simulink model "PVESsystem"  (R2024a)
settings: Solver=FixedStepDiscrete  StartTime=0.0  StopTime=4  FixedStep=1e-7  MaxStep=1e-6  RelTol=1e-3
libraries: spsSeriesRLCBranchLib x11, spsMultimeterLib x4, spsDiodeLib x2, spsMosfetLib x2, slpidlib x2, eePwmGenerator x2, spsVoltageMeasurementLib x2, spsCurrentMeasurementLib x1, spsDCVoltageSourceLib x1, spsPVArrayLib x1, sps_lib x1
settings Model: Creator=admin  LastModifiedBy=ZE
settings SolverCC: AllowMultiTaskInputOutput=on
settings ModelReferenceCC: EnableParallelModelReferenceBuilds=on
settings SFSimCC: SimTargetLang=C++  GPUAcceleration=on  SimDLTargetLibrary=cudnn

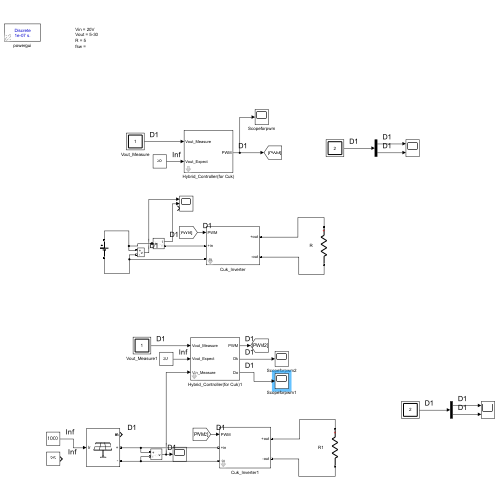
[thumbnail: Simulink's stored preview of the top-level diagram]
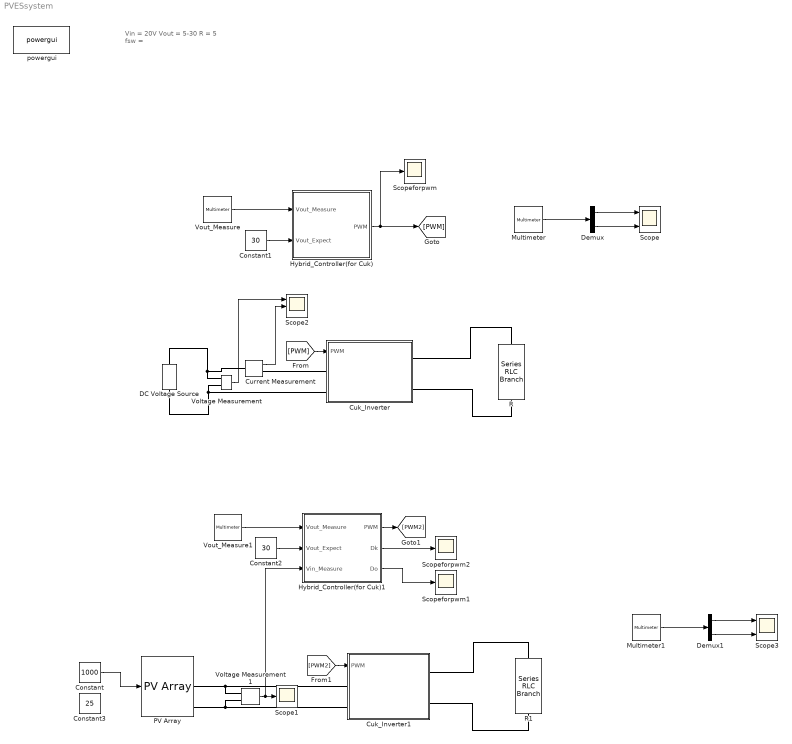
== system PVESsystem ==
  note: Vin = 20V
      | Vout = 5-30
      | R = 5
      | fsw =
  Constant : Constant  Value=1000
  Constant1 : Constant  Value=30
  Constant2 : Constant  Value=30
  Constant3 : Constant  Value=25
  Cuk_Inverter : Subsystem  mask{Vin=30, Vout_Expect=40, Fsw=100e3, detaIL1=0.1, detaIL2=0.1, detaUC1=0.1, detaUC2=0.1}
      mask prompts: Fsw "Switch Frequency"; detaIL1 "电感纹波"; detaIL2 "电感纹波"; detaUC1 "电压纹波"; detaUC2 "电压纹波"
      mask DialogControl ParameterGroupVar Prompt: 参数
  Cuk_Inverter1 : Subsystem  mask{Vin=30, Vout_Expect=40, Fsw=100e3, detaIL1=0.1, detaIL2=0.1, detaUC1=0.1, detaUC2=0.1}
      mask prompts: Fsw "Switch Frequency"; detaIL1 "电感纹波"; detaIL2 "电感纹波"; detaUC1 "电压纹波"; detaUC2 "电压纹波"
      mask DialogControl ParameterGroupVar Prompt: 参数
  Current Measurement : spsCurrentMeasurementLib/Current Measurement  PhasorSimulation=off  OutputType=Complex  PSBequivalent=0
  DC Voltage Source : spsDCVoltageSourceLib/DC Voltage Source  Amplitude=30  Measurements=None
  Demux : Demux  Outputs=2
  Demux1 : Demux  Outputs=2
  Hybrid_Controller(for Cuk) : Subsystem  mask{Vout_Expect=20, Vin=30, Fsw=100e3}
      mask prompts: Fsw "switch frequency"
      mask DialogControl ParameterGroupVar Prompt: 参数
  Hybrid_Controller(for Cuk)1 : Subsystem  mask{Vout_Expect=20, Vin=30, Fsw=100e3}
      mask prompts: Fsw "switch frequency"
      mask DialogControl ParameterGroupVar Prompt: 参数
  Multimeter : spsMultimeterLib/Multimeter  L=4  sel=[1 3]  yselected={}  Gain=[1 1]  OutputType=Complex  PlotAtSimulationStop=off  PhasorSimulation=off
  Multimeter1 : spsMultimeterLib/Multimeter  L=4  sel=[2 4]  yselected={}  Gain=[1 1]  OutputType=Complex  PlotAtSimulationStop=off  PhasorSimulation=off
  PV Array : spsPVArrayLib/PV Array  Npar=20  Nser=1  PlotType=array @ 1000 W/m2 & specified temperatures  S_vec="[ 1000  500  100 ]"  Temp_C_vec="[ 45 25  ]"  ModuleName=User-defined  PlotWhenSelected=off  Pm=213.15  Ncell=60  Voc=36.3  Isc=7.84  Vm=29  Im=7.35  beta_Voc_pc=-0.36099  alpha_Isc_pc=0.102  beta_Voc=-0.13104  alpha_Isc=0.0079968  IL=7.8654  I0=2.9273e-10  nI=0.98119  Rsh=313.0553  Rs=0.39381  RobustModel=on  RobustCellTemperature=25  BAL=on  Tc=1e-6  Tfilter=5e-5
  R : spsSeriesRLCBranchLib/Series RLC Branch  LConnTagsString=__new0  RConnTagsString=__new0  BranchType=R  Resistance=5  Inductance=1e-3  SetiL0=off  InitialCurrent=0  Capacitance=1e-6  Setx0=off  InitialVoltage=0  Measurements=Branch voltage and current
  R1 : spsSeriesRLCBranchLib/Series RLC Branch  LConnTagsString=__new0  RConnTagsString=__new0  BranchType=R  Resistance=5  Inductance=1e-3  SetiL0=off  InitialCurrent=0  Capacitance=1e-6  Setx0=off  InitialVoltage=0  Measurements=Branch voltage and current
  Scope : Scope  NumInputPorts=2
  Scope1 : Scope
  Scope2 : Scope  NumInputPorts=3
  Scope3 : Scope  NumInputPorts=2
  Scopeforpwm : Scope
  Scopeforpwm1 : Scope
  Scopeforpwm2 : Scope
  Voltage Measurement : spsVoltageMeasurementLib/Voltage Measurement  PhasorSimulation=off  OutputType=Complex  PSBequivalent=0
  Voltage Measurement1 : spsVoltageMeasurementLib/Voltage Measurement  PhasorSimulation=off  OutputType=Complex  PSBequivalent=0
  Vout_Measure : spsMultimeterLib/Multimeter  L=4  sel=1  yselected={}  Gain=1  OutputType=Complex  PlotAtSimulationStop=off  PhasorSimulation=off
  Vout_Measure1 : spsMultimeterLib/Multimeter  L=4  sel=2  yselected={}  Gain=1  OutputType=Complex  PlotAtSimulationStop=off  PhasorSimulation=off
  powergui : sps_lib/powergui  Priority=1  SimulationMode=Discrete  SampleTime=1e-7  frequency=60  Iterations=50  frequencyindice=0  Pbase=100e6  ErrMax=1e-4  UnitsV=kV  UnitsW=MW  buscounter=0  FunctionMessages=off  echomessages=off  EnableUseOfTLC=off  CurrentSourceSwitches=off  DisableSnubberDevices=off  DisableRonSwitches=off  DisableVfSwitches=off  DisplayEquations=off  AutomaticDiscreteSolvers=off  SolverType=Tustin/Backward Euler (TBE)  Interpol=off  ExternalGateDelay=off  methode=off  Ts=100  x0status=blocks  SPID=on  SwTol=0  HookPort=off  NonlinearTolerance=1e-4  nMaxIteration=100  ContinueOnMaxIteration=off  RestoreLinks=warning  ResistiveCurrentMeasurement=off  Frange=[0:2:500]  Ylog=off  Xlog=on  ShowGrid=off  save=off  variable=ZData  structure=0  ZoomFFT=off  StartTime=0.0  cycles=1  DisplayStyle=1  fundamental=60  FreqAxis=off  MaxFrequency=1000  frequencyindicesteady=1  RmsSteady=1  display=off
  wires:
  Vout_Measure/1 -> Hybrid_Controller(for Cuk)/1(Vout_Measure)
  Hybrid_Controller(for Cuk)/1(PWM) -> Scopeforpwm/1, [PWM]
  [PWM] -> Cuk_Inverter/1(PWM)
  Voltage Measurement/1 -> Scope2/1
  Current Measurement/1 -> Scope2/2
  Constant1/1 -> Hybrid_Controller(for Cuk)/2(Vout_Expect)
  Multimeter/1 -> Demux/1
  Demux/1 -> Scope/1
  Demux/2 -> Scope/2
  [PWM2] -> Cuk_Inverter1/1(PWM)
  Constant2/1 -> Hybrid_Controller(for Cuk)1/2(Vout_Expect)
  Vout_Measure1/1 -> Hybrid_Controller(for Cuk)1/1(Vout_Measure)
  Hybrid_Controller(for Cuk)1/1(PWM) -> [PWM2]
  Demux1/2 -> Scope3/2
  Demux1/1 -> Scope3/1
  Multimeter1/1 -> Demux1/1
  Constant/1 -> PV Array/1
  Voltage Measurement1/1 -> Hybrid_Controller(for Cuk)1/3(Vin_Measure), Scope1/1
  Hybrid_Controller(for Cuk)1/2(Dk) -> Scopeforpwm2/1
  Hybrid_Controller(for Cuk)1/3(Do) -> Scopeforpwm1/1
  connections:
  R/LConn1 -- Cuk_Inverter/RConn1
  R/RConn1 -- Cuk_Inverter/RConn2
  Current Measurement/LConn1 -- DC Voltage Source/RConn1 -- Voltage Measurement/LConn1
  Voltage Measurement/LConn2 -- DC Voltage Source/LConn1 -- Cuk_Inverter/LConn2
  Current Measurement/RConn1 -- Cuk_Inverter/LConn1
  Cuk_Inverter1/LConn1 -- Voltage Measurement1/LConn1 -- PV Array/RConn1
  PV Array/RConn2 -- Voltage Measurement1/LConn2 -- Cuk_Inverter1/LConn2
  R1/RConn1 -- Cuk_Inverter1/RConn2
  R1/LConn1 -- Cuk_Inverter1/RConn1

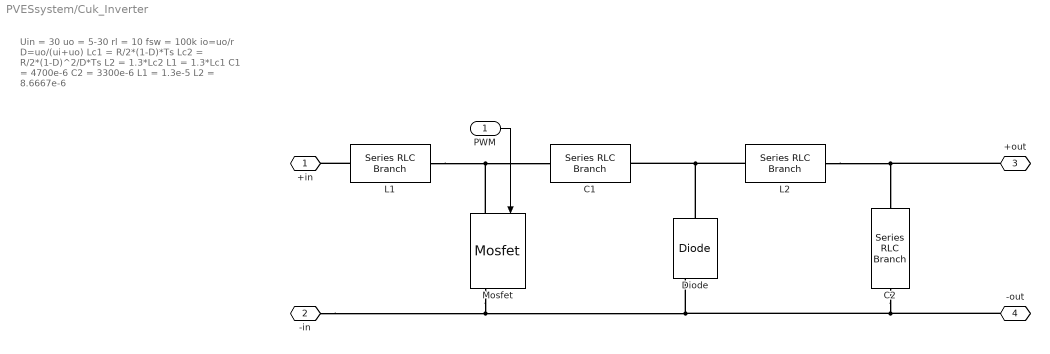
== system PVESsystem/Cuk_Inverter ==
  note: Uin = 30
      | uo = 5-30
      | rl = 10
      | fsw = 100k
      | io=uo/r
      |
      | D=uo/(ui+uo)
      | Lc1 = R/2*(1-D)*Ts
      | Lc2 = R/2*(1-D)^2/D*Ts
      | L2 = 1.3*Lc2
      | L1 = 1.3*Lc1
      | C1 = 4700e-6
      | C2 = 3300e-6
      |
      | L1 = 1.3e-5
      | L2 = 8.6667e-6
  PWM : Inport
  C1 : spsSeriesRLCBranchLib/Series RLC Branch  LConnTagsString=__new0  RConnTagsString=__new0  BranchType=C  Resistance=1  Inductance=1e-3  SetiL0=off  InitialCurrent=0  Capacitance=0.0047  Setx0=off  InitialVoltage=0  Measurements=None
  C2 : spsSeriesRLCBranchLib/Series RLC Branch  LConnTagsString=__new0  RConnTagsString=__new0  BranchType=C  Resistance=1  Inductance=1e-3  SetiL0=off  InitialCurrent=0  Capacitance=0.0033  Setx0=off  InitialVoltage=0  Measurements=None
  Diode : spsDiodeLib/Diode  Ron=0.001  Lon=0  Vf=0.8  IC=0  UseSnubber=0  Rs=500  Cs=250e-9  Measurements=on
  L1 : spsSeriesRLCBranchLib/Series RLC Branch  LConnTagsString=__new0  RConnTagsString=__new0  BranchType=L  Resistance=1  Inductance=1.3e-5  SetiL0=off  InitialCurrent=0  Capacitance=1e-6  Setx0=off  InitialVoltage=0  Measurements=None
  L2 : spsSeriesRLCBranchLib/Series RLC Branch  LConnTagsString=__new0  RConnTagsString=__new0  BranchType=L  Resistance=1  Inductance=8.6667e-6  SetiL0=off  InitialCurrent=0  Capacitance=1e-6  Setx0=off  InitialVoltage=0  Measurements=None
  Mosfet : spsMosfetLib/Mosfet  Ron=0.1  Lon=0  Rd=0.01  Vfd=0  IC=0  Rs=1e5  Cs=inf  Measurements=on
  +in : PMIOPort  Side=Left
  -in : PMIOPort  Port=2  Side=Left
  +out : PMIOPort  Port=3  Side=Right
  -out : PMIOPort  Port=4  Side=Right
  wires:
  PWM/1 -> Mosfet/1
  connections:
  L2/RConn1 -- +out/RConn1 -- C2/LConn1
  L2/LConn1 -- Diode/LConn1 -- C1/RConn1
  L1/LConn1 -- +in/RConn1
  L1/RConn1 -- Mosfet/LConn1 -- C1/LConn1
  Mosfet/RConn1 -- -in/RConn1 -- -out/RConn1 -- C2/RConn1 -- Diode/RConn1

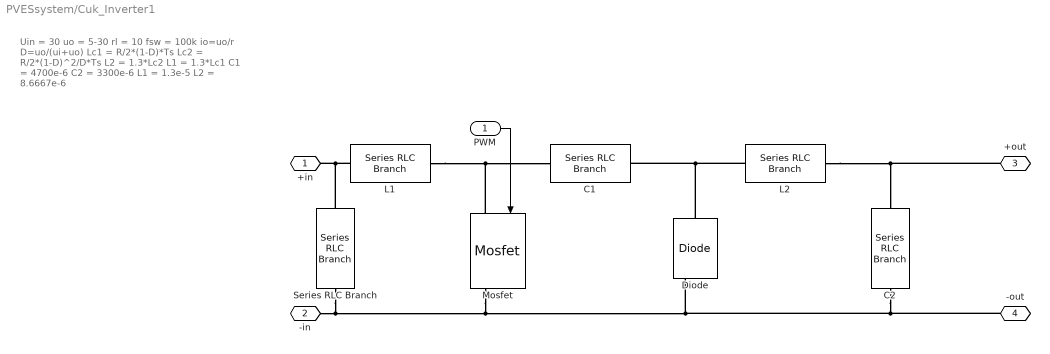
== system PVESsystem/Cuk_Inverter1 ==
  note: Uin = 30
      | uo = 5-30
      | rl = 10
      | fsw = 100k
      | io=uo/r
      |
      | D=uo/(ui+uo)
      | Lc1 = R/2*(1-D)*Ts
      | Lc2 = R/2*(1-D)^2/D*Ts
      | L2 = 1.3*Lc2
      | L1 = 1.3*Lc1
      | C1 = 4700e-6
      | C2 = 3300e-6
      |
      | L1 = 1.3e-5
      | L2 = 8.6667e-6
  PWM : Inport
  C1 : spsSeriesRLCBranchLib/Series RLC Branch  LConnTagsString=__new0  RConnTagsString=__new0  BranchType=C  Resistance=1  Inductance=1e-3  SetiL0=off  InitialCurrent=0  Capacitance=0.0047  Setx0=off  InitialVoltage=0  Measurements=None
  C2 : spsSeriesRLCBranchLib/Series RLC Branch  LConnTagsString=__new0  RConnTagsString=__new0  BranchType=C  Resistance=1  Inductance=1e-3  SetiL0=off  InitialCurrent=0  Capacitance=0.0033  Setx0=off  InitialVoltage=0  Measurements=None
  Diode : spsDiodeLib/Diode  Ron=0.001  Lon=0  Vf=0.8  IC=0  UseSnubber=0  Rs=500  Cs=250e-9  Measurements=on
  L1 : spsSeriesRLCBranchLib/Series RLC Branch  LConnTagsString=__new0  RConnTagsString=__new0  BranchType=L  Resistance=1  Inductance=1.3e-5  SetiL0=off  InitialCurrent=0  Capacitance=1e-6  Setx0=off  InitialVoltage=0  Measurements=None
  L2 : spsSeriesRLCBranchLib/Series RLC Branch  LConnTagsString=__new0  RConnTagsString=__new0  BranchType=L  Resistance=1  Inductance=8.6667e-6  SetiL0=off  InitialCurrent=0  Capacitance=1e-6  Setx0=off  InitialVoltage=0  Measurements=None
  Mosfet : spsMosfetLib/Mosfet  Ron=0.1  Lon=0  Rd=0.01  Vfd=0  IC=0  Rs=1e5  Cs=inf  Measurements=on
  Series RLC Branch : spsSeriesRLCBranchLib/Series RLC Branch  LConnTagsString=__new0  RConnTagsString=__new0  BranchType=C  Resistance=1  Inductance=1e-3  SetiL0=off  InitialCurrent=0  Capacitance=1e-6  Setx0=off  InitialVoltage=0  Measurements=None
  +in : PMIOPort  Side=Left
  -in : PMIOPort  Port=2  Side=Left
  +out : PMIOPort  Port=3  Side=Right
  -out : PMIOPort  Port=4  Side=Right
  wires:
  PWM/1 -> Mosfet/1
  connections:
  L2/RConn1 -- +out/RConn1 -- C2/LConn1
  L2/LConn1 -- Diode/LConn1 -- C1/RConn1
  L1/LConn1 -- Series RLC Branch/LConn1 -- +in/RConn1
  L1/RConn1 -- Mosfet/LConn1 -- C1/LConn1
  Mosfet/RConn1 -- -in/RConn1 -- Series RLC Branch/RConn1 -- -out/RConn1 -- C2/RConn1 -- Diode/RConn1

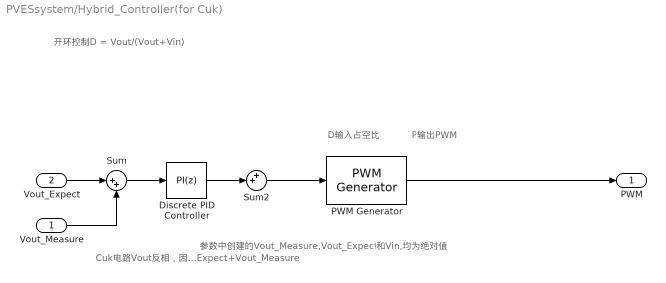
== system PVESsystem/Hybrid_Controller(for Cuk) ==
  note: 开环控制D = Vout/(Vout+Vin)
  note: 参数中创建的Vout_Measure,Vout_Expect和Vin,均为绝对值
  note: Cuk电路Vout反相，因此这里设置为Vout_Expect+Vout_Measure
  note: P输出PWM
  note: D输入占空比
  Vout_Measure : Inport
  Vout_Expect : Inport  Port=2
  Discrete PID Controller : slpidlib/PID Controller  Controller=PI  Form=Parallel  TimeDomain=Discrete-time  UseExternalTs=off  SampleTime=-1  IntegratorMethod=Forward Euler  FilterMethod=Forward Euler  ControllerParametersSource=internal  P=(1/(Vin+1))*10  I=(1/(Vin+1))*5*20  UseKiTs=off  D=0  UseExternalDerivativeSource=off  N=100  UseFilter=on  TunerSelectOption=Transfer Function Based (PID Tuner App)  InitialConditionSource=internal  InitialConditionForIntegrator=0  InitialConditionForFilter=0  DifferentiatorICPrevScaledInput=0  ExternalReset=none  TrackingMode=off  Kt=1  LimitOutput=on  SatLimitsSource=internal  UpperSaturationLimit=0.98  LowerSaturationLimit=0  LinearizeAsGain=off  AntiWindupMode=none  Kb=1  LimitIntegrator=off  UpperIntegratorSaturationLimit=inf  LowerIntegratorSaturationLimit=-inf  POutMin=[]  POutMax=[]  IOutMin=[]  IOutMax=[]  DOutMin=[]  DOutMax=[]  NOutMin=[]  NOutMax=[]  SumOutMin=[]  SumOutMax=[]  SaturationOutMin=[]  SaturationOutMax=[]  PParamMin=[]  PParamMax=[]  IParamMin=[]  IParamMax=[]  DParamMin=[]  DParamMax=[]  NParamMin=[]  NParamMax=[]  KbParamMin=[]  KbParamMax=[]  KtParamMin=[]  KtParamMax=[]  KbOutMin=[]  KbOutMax=[]  KtOutMin=[]  KtOutMax=[]  IntegratorOutMin=[]  IntegratorOutMax=[]  FilterOutMin=[]  FilterOutMax=[]  SumI1OutMin=[]  SumI1OutMax=[]  SumI2OutMin=[]  SumI2OutMax=[]  SumI3OutMin=[]  SumI3OutMax=[]  SumI4OutMin=[]  SumI4OutMax=[]  SumDOutMin=[]  SumDOutMax=[]  DifferentiatorOutMin=[]  DifferentiatorOutMax=[]  FilterDiffOutCoefMin=[]  FilterDiffOutCoefMax=[]  ReciprocalOutMin=[]  ReciprocalOutMax=[]  SumDenOutMin=[]  SumDenOutMax=[]  SumNumOutMin=[]  SumNumOutMax=[]  DivideOutMin=[]  DivideOutMax=[]  UdiffTsProdOutMin=[]  UdiffTsProdOutMax=[]  NTsProdOutMin=[]  NTsProdOutMax=[]  UintegralTsProdOutMin=[]  UintegralTsProdOutMax=[]  UngainTsProdOutMin=[]  UngainTsProdOutMax=[]  ClampingZeroOutDataTypeStr=Inherit: Inherit via back propagation  ClampingZeroOutMin=[]  ClampingZeroOutMax=[]  FilterDenConstantOutDataTypeStr=Inherit: Inherit via back propagation  FilterDenConstantOutMin=[]  FilterDenConstantOutMax=[]  PCopyOutDataTypeStr=Inherit: Inherit via back propagation  PCopyOutMin=[]  PCopyOutMax=[]  NCopyOutDataTypeStr=Inherit: Inherit via back propagation  NCopyOutMin=[]  NCopyOutMax=[]  IntegratorContinuousStateAttributes=''  IntegratorStateMustResolveToSignalObject=off  IntegratorRTWStateStorageClass=Auto  FilterContinuousStateAttributes=''  FilterStateMustResolveToSignalObject=off  FilterRTWStateStorageClass=Auto  ParallelPVariant=InternalParameters  IdealPVariant=Disabled  IVariant=InternalParameters  DVariant=Disabled  IntegratorVariant=Discrete  SatVariant=Enabled  AWVariant=Passthrough  PCopyVariant=Disabled  TRVariant=Disabled  FdbkBlocksVariant=Forward  IdealPFdbkVariant=Disabled  SatFdbkVariant=Disabled  DerivativeFilterVariant=Disabled  NVariant=Disabled  NCopyVariant=Disabled_SignalSpec  FilterICVariant=Disabled  IntegratorICVariant=InternalICs  ExternalResetVariant=Disabled  TRSumVariant=Passthrough  SumFdbkVariant=Disabled  SumVariant=Sum_PI  TsampFilterVariant=InternalTs  TsampNgainVariant=Passthrough  TsampIntegralVariant=Disabled_SignalSpec  ExternalSaturationOutDataTypeStr=Inherit: Same as second input  DerivativeSourceVariant=Disabled
      settings: LibrarySourceBlock=simulink/Discrete/Discrete PID Controller
  PWM Generator : eePwmGenerator/PWM Generator  CarrCount=Up  Tper=1e-5  Tdelay=0  Ts=1e-7
  Sum : Sum  Inputs=|++
  Sum2 : Sum  Inputs=++|
  PWM : Outport
  wires:
  Sum/1 -> Discrete PID Controller/1
  PWM Generator/1 -> PWM/1
  Vout_Expect/1 -> Sum/1
  Vout_Measure/1 -> Sum/2
  Discrete PID Controller/1 -> Sum2/2
  Sum2/1 -> PWM Generator/1

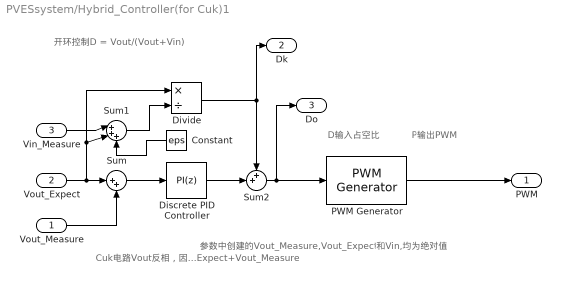
== system PVESsystem/Hybrid_Controller(for Cuk)1 ==
  note: 开环控制D = Vout/(Vout+Vin)
  note: 参数中创建的Vout_Measure,Vout_Expect和Vin,均为绝对值
  note: Cuk电路Vout反相，因此这里设置为Vout_Expect+Vout_Measure
  note: P输出PWM
  note: D输入占空比
  Vout_Measure : Inport
  Vout_Expect : Inport  Port=2
  Vin_Measure : Inport  Port=3
  Constant : Constant  Value=eps
  Discrete PID Controller : slpidlib/PID Controller  Controller=PI  Form=Parallel  TimeDomain=Discrete-time  UseExternalTs=off  SampleTime=-1  IntegratorMethod=Forward Euler  FilterMethod=Forward Euler  ControllerParametersSource=internal  P=(1/(Vin+1))*10  I=(1/(Vin+1))*5*20  UseKiTs=off  D=0  UseExternalDerivativeSource=off  N=100  UseFilter=on  TunerSelectOption=Transfer Function Based (PID Tuner App)  InitialConditionSource=internal  InitialConditionForIntegrator=0  InitialConditionForFilter=0  DifferentiatorICPrevScaledInput=0  ExternalReset=none  TrackingMode=off  Kt=1  LimitOutput=on  SatLimitsSource=internal  UpperSaturationLimit=0.3  LowerSaturationLimit=-0.3  LinearizeAsGain=off  AntiWindupMode=none  Kb=1  LimitIntegrator=off  UpperIntegratorSaturationLimit=inf  LowerIntegratorSaturationLimit=-inf  POutMin=[]  POutMax=[]  IOutMin=[]  IOutMax=[]  DOutMin=[]  DOutMax=[]  NOutMin=[]  NOutMax=[]  SumOutMin=[]  SumOutMax=[]  SaturationOutMin=[]  SaturationOutMax=[]  PParamMin=[]  PParamMax=[]  IParamMin=[]  IParamMax=[]  DParamMin=[]  DParamMax=[]  NParamMin=[]  NParamMax=[]  KbParamMin=[]  KbParamMax=[]  KtParamMin=[]  KtParamMax=[]  KbOutMin=[]  KbOutMax=[]  KtOutMin=[]  KtOutMax=[]  IntegratorOutMin=[]  IntegratorOutMax=[]  FilterOutMin=[]  FilterOutMax=[]  SumI1OutMin=[]  SumI1OutMax=[]  SumI2OutMin=[]  SumI2OutMax=[]  SumI3OutMin=[]  SumI3OutMax=[]  SumI4OutMin=[]  SumI4OutMax=[]  SumDOutMin=[]  SumDOutMax=[]  DifferentiatorOutMin=[]  DifferentiatorOutMax=[]  FilterDiffOutCoefMin=[]  FilterDiffOutCoefMax=[]  ReciprocalOutMin=[]  ReciprocalOutMax=[]  SumDenOutMin=[]  SumDenOutMax=[]  SumNumOutMin=[]  SumNumOutMax=[]  DivideOutMin=[]  DivideOutMax=[]  UdiffTsProdOutMin=[]  UdiffTsProdOutMax=[]  NTsProdOutMin=[]  NTsProdOutMax=[]  UintegralTsProdOutMin=[]  UintegralTsProdOutMax=[]  UngainTsProdOutMin=[]  UngainTsProdOutMax=[]  ClampingZeroOutDataTypeStr=Inherit: Inherit via back propagation  ClampingZeroOutMin=[]  ClampingZeroOutMax=[]  FilterDenConstantOutDataTypeStr=Inherit: Inherit via back propagation  FilterDenConstantOutMin=[]  FilterDenConstantOutMax=[]  PCopyOutDataTypeStr=Inherit: Inherit via back propagation  PCopyOutMin=[]  PCopyOutMax=[]  NCopyOutDataTypeStr=Inherit: Inherit via back propagation  NCopyOutMin=[]  NCopyOutMax=[]  IntegratorContinuousStateAttributes=''  IntegratorStateMustResolveToSignalObject=off  IntegratorRTWStateStorageClass=Auto  FilterContinuousStateAttributes=''  FilterStateMustResolveToSignalObject=off  FilterRTWStateStorageClass=Auto  ParallelPVariant=InternalParameters  IdealPVariant=Disabled  IVariant=InternalParameters  DVariant=Disabled  IntegratorVariant=Discrete  SatVariant=Enabled  AWVariant=Passthrough  PCopyVariant=Disabled  TRVariant=Disabled  FdbkBlocksVariant=Forward  IdealPFdbkVariant=Disabled  SatFdbkVariant=Disabled  DerivativeFilterVariant=Disabled  NVariant=Disabled  NCopyVariant=Disabled_SignalSpec  FilterICVariant=Disabled  IntegratorICVariant=InternalICs  ExternalResetVariant=Disabled  TRSumVariant=Passthrough  SumFdbkVariant=Disabled  SumVariant=Sum_PI  TsampFilterVariant=InternalTs  TsampNgainVariant=Passthrough  TsampIntegralVariant=Disabled_SignalSpec  ExternalSaturationOutDataTypeStr=Inherit: Same as second input  DerivativeSourceVariant=Disabled
      settings: LibrarySourceBlock=simulink/Discrete/Discrete PID Controller
  Divide : Product  Inputs=*/
  PWM Generator : eePwmGenerator/PWM Generator  CarrCount=Up  Tper=1e-5  Tdelay=0  Ts=1e-7
  Sum : Sum  Inputs=|++
  Sum1 : Sum  Inputs=|+++
  Sum2 : Sum  Inputs=++|
  PWM : Outport
  Dk : Outport  Port=2
  Do : Outport  Port=3
  wires:
  Sum/1 -> Discrete PID Controller/1
  PWM Generator/1 -> PWM/1
  Vout_Expect/1 -> Divide/1, Sum1/2, Sum/1
  Vout_Measure/1 -> Sum/2
  Discrete PID Controller/1 -> Sum2/2
  Sum2/1 -> Do/1, PWM Generator/1
  Sum1/1 -> Divide/2
  Vin_Measure/1 -> Sum1/1
  Constant/1 -> Sum1/3
  Divide/1 -> Dk/1, Sum2/1
